simulink model "5kW_singlephase_grid-connected inverter_"  (R2020b)
settings: Solver=FixedStepDiscrete  StartTime=0.0  StopTime=10  FixedStep=1e-6  RelTol=1e-3
undefined symbols (not defined in the file): sigbuilder_block
libraries: powerlib x17, simulink x2, pid_lib x2, re_lib x1, powerlib_meascontrol x1
settings Model: SimulationMode=accelerator  Creator=zhaoy  LastModifiedBy=gc45
settings DataIOCC: ReturnWorkspaceOutputs=off
settings OptimizationCC: LifeSpan=inf
settings DebuggingCC: ArithmeticOperatorsInVariantConditions=warning
settings SFSimCC: SimUseLocalCustomCode=off  CustomCodeUndefinedFunction=UseInterfaceOnly
settings RTWCC: RTWUseLocalCustomCode=off
settings CodeAppCC: StateflowObjectComments=on
settings SimscapeCC: SimscapeNormalizeSystem=off

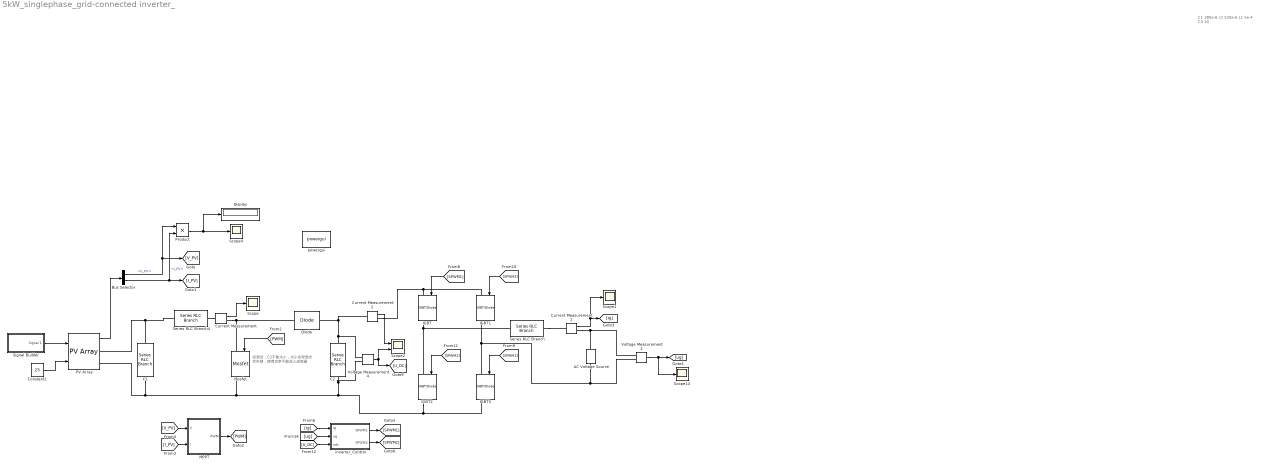
== system 5kW_singlephase_grid-connected inverter_ ==
  note: C1 380e-6
      | c2 520e-6
      | L1 5e-4
      | C3 20
  note: 经测试，C2不能太小，太小会导致光
      | 伏失稳，使得功率不能流入逆变器
  AC Voltage Source : powerlib/Electrical Sources/AC Voltage Source  Amplitude=311  Phase=180  Frequency=50  SampleTime=0  Measurements=None  BusType=swing  Pref=10e3  Qref=0  Qmin=-inf  Qmax=+inf
  Bus Selector : BusSelector  OutputSignals=V_PV,I_PV
  C1 : powerlib/Elements/Series RLC Branch  LConnTagsString=__new0  RConnTagsString=__new0  BranchType=C  Resistance=1  Inductance=3.05e-3  SetiL0=off  InitialCurrent=0  Capacitance=10e-6  Setx0=off  InitialVoltage=0  Measurements=Branch voltage
  C2 : powerlib/Elements/Series RLC Branch  LConnTagsString=__new0  RConnTagsString=__new0  BranchType=C  Resistance=1  Inductance=3.05e-3  SetiL0=off  InitialCurrent=0  Capacitance=6e-3  Setx0=off  InitialVoltage=0  Measurements=Branch voltage
  Constant1 : Constant  Value=25
  Current Measurement : powerlib/Measurements/Current Measurement  PhasorSimulation=off  OutputType=Complex  PSBequivalent=0
  Current Measurement1 : powerlib/Measurements/Current Measurement  PhasorSimulation=off  OutputType=Complex  PSBequivalent=0
  Current Measurement2 : powerlib/Measurements/Current Measurement  PhasorSimulation=off  OutputType=Complex  PSBequivalent=0
  Diode : powerlib/Power Electronics/Diode  Ron=0.001  Lon=0  Vf=0.8  IC=0  UseSnubber=off  Rs=500  Cs=250e-9  Measurements=off
  Display : Display
  IGBT{,1..3} (4 alike) : powerlib/Power Electronics/IGBT//Diode  Ron=1e-3  Rs=1e5  Cs=inf  Measurements=on
  MPPT : Subsystem
  Mosfet : powerlib/Power Electronics/Mosfet  Ron=0.1  Lon=0  Rd=0.01  Vfd=0  IC=0  Rs=1e5  Cs=inf  Measurements=on
  PV Array : re_lib/Solar/PV Array  Npar=2  Nser=7  PlotType=array @ 25 deg.C & specified irradiances  S_vec=[2000 1500 1000 ]  Temp_C_vec="[ 45 25  ]"  ModuleName=User-defined  PlotWhenSelected=off  Pm=213.15  Ncell=60  Voc=36.3  Isc=7.84  Vm=29  Im=7.35  beta_Voc_pc=-0.36099  alpha_Isc_pc=0.102  beta_Voc=-0.13104  alpha_Isc=0.0079968  IL=7.8654  I0=2.9273e-10  nI=0.98119  Rsh=313.0553  Rs=0.39381  RobustModel=off  RobustCellTemperature=313.3991  BAL=on  Tc=1e-6  Tfilter=5e-5
  Product : Product
  Scope{,1,4,14} (4 alike) : Scope
  Scope2 : Scope  NumInputPorts=2
  Series RLC Branch : powerlib/Elements/Series RLC Branch  LConnTagsString=__new0  RConnTagsString=__new0  BranchType=RL  Resistance=0.01  Inductance=20e-3  SetiL0=off  InitialCurrent=0  Capacitance=1e-6  Setx0=off  InitialVoltage=0  Measurements=None
  Series RLC Branch4 : powerlib/Elements/Series RLC Branch  LConnTagsString=__new0  RConnTagsString=__new0  BranchType=L  Resistance=1  Inductance=2.65e-3  SetiL0=off  InitialCurrent=0  Capacitance=1e-6  Setx0=off  InitialVoltage=0  Measurements=None
  Signal Builder : Subsystem  Tag=STV Subsys  LoadFcn=sigbuilder_block('load');  StartFcn=sigbuilder_block('start');  StopFcn=sigbuilder_block('stop');  ClipboardFcn=sigbuilder_block('clipboard');  mask(Sigbuilder block){tuvar=[0:10]}
      mask help: Simulink:masks:SigbuilderBlock_MD
      mask init:
      | if ~strcmp(get_param(bdroot(gcbh),'SimulationStatus'),'stopped') tuvar = sigbuilder_block('maskInit'); end
      settings: CopyFcn=sigbuilder_block('copy');  DeleteFcn=sigbuilder_block('delete');  ModelCloseFcn=sigbuilder_block('modelClose');  PreSaveFcn=sigbuilder_block('preSave');  PauseFcn=sigbuilder_block('pause');  ContinueFcn=sigbuilder_block('continue');  NameChangeFcn=sigbuilder_block('namechange');  OpenFcn=sigbuilder_block('open',[437.6 199.2 550.4 400 ]);  CloseFcn=sigbuilder_block('close');
      mask Display: plot(0, 0, 100, 100,[2, 2, 32, 32, 2], [68, 8, 8, 68, 68],[32, 2], [38, 38], [32, 19, 2],[53, 60, 44], [32, 17, 17, 2],[16, 16, 31, 31]);txt = getActiveGroup(gcbh);text(2, 100, txt,'verticalAlignment', 'top');
  Voltage Measurement2 : powerlib/Measurements/Voltage Measurement  PhasorSimulation=off  OutputType=Complex  PSBequivalent=0
  Voltage Measurement4 : powerlib/Measurements/Voltage Measurement  PhasorSimulation=off  OutputType=Complex  PSBequivalent=0
  inverter_Control : Subsystem
  powergui : powerlib/powergui  Priority=1  SimulationMode=Discrete  SampleTime=1e-6  frequency=50  Iterations=50  frequencyindice=0  Pbase=100e6  ErrMax=1e-4  UnitsV=kV  UnitsW=MW  buscounter=0  FunctionMessages=off  echomessages=off  EnableUseOfTLC=off  CurrentSourceSwitches=off  DisableSnubberDevices=off  DisableRonSwitches=off  DisableVfSwitches=off  DisplayEquations=off  AutomaticDiscreteSolvers=off  SolverType=Tustin/Backward Euler (TBE)  Interpol=off  ExternalGateDelay=off  methode=off  Ts=10  x0status=blocks  SPID=off  SwTol=0  HookPort=off  NonlinearTolerance=1e-4  nMaxIteration=100  ContinueOnMaxIteration=off  RestoreLinks=warning  ResistiveCurrentMeasurement=off  Frange=[0:2:500]  Ylog=off  Xlog=on  ShowGrid=off  save=off  variable=ZData  structure=Udc_pv  ZoomFFT=off  StartTime=8  cycles=20  DisplayStyle=1  fundamental=50  FreqAxis=on  MaxFrequency=500  frequencyindicesteady=1  RmsSteady=2  display=off
  wires:
  PV Array/1 -> Bus Selector/1
  [PWM] -> Mosfet/1
  Signal Builder/1(Signal 1) -> PV Array/1
  Constant1/1 -> PV Array/2
  Bus Selector/1 -> Product/1, [V_PV]  "<V_PV>"
  Bus Selector/2 -> Product/2, [I_PV]  "<I_PV>"
  Product/1 -> Display/1, Scope4/1
  [V_PV] -> MPPT/1(V)
  [I_PV] -> MPPT/2(I)
  MPPT/1(PWM) -> [PWM]
  Current Measurement1/1 -> Scope1/1, [ig]
  Voltage Measurement2/1 -> Scope14/1, [ug]
  [SPWM1] -> IGBT/1
  [SPWM1] -> IGBT3/1
  [SPWM2] -> IGBT1/1
  [SPWM2] -> IGBT2/1
  Current Measurement/1 -> Scope/1
  Voltage Measurement4/1 -> Scope2/2, [U_DC]
  Current Measurement2/1 -> Scope2/1
  [ig] -> inverter_Control/1(Ig)
  [ug] -> inverter_Control/2(ug)
  [U_DC] -> inverter_Control/3(udc)
  inverter_Control/1(SPWM1) -> [SPWM1]
  inverter_Control/2(SPWM2) -> [SPWM2]
  connections:
  IGBT2/LConn1 -- Series RLC Branch/LConn1 -- IGBT/RConn1
  IGBT3/LConn1 -- IGBT1/RConn1 -- Voltage Measurement2/LConn2 -- AC Voltage Source/RConn1
  Current Measurement/RConn1 -- Mosfet/LConn1 -- Diode/LConn1
  C1/LConn1 -- Series RLC Branch4/LConn1 -- PV Array/RConn1
  IGBT2/RConn1 -- PV Array/RConn2 -- C1/RConn1 -- Mosfet/RConn1 -- Voltage Measurement4/LConn2 -- C2/RConn1 -- IGBT3/RConn1
  Current Measurement1/RConn1 -- Voltage Measurement2/LConn1 -- AC Voltage Source/LConn1
  Series RLC Branch4/RConn1 -- Current Measurement/LConn1
  Series RLC Branch/RConn1 -- Current Measurement1/LConn1
  Voltage Measurement4/LConn1 -- Current Measurement2/LConn1 -- Diode/RConn1 -- C2/LConn1
  IGBT1/LConn1 -- Current Measurement2/RConn1 -- IGBT/LConn1

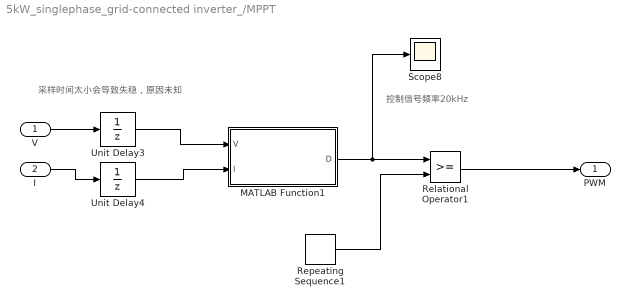
== system 5kW_singlephase_grid-connected inverter_/MPPT ==
  note: 采样时间太小会导致失稳，原因未知
  note: 控制信号频率20kHz
  V : Inport
  I : Inport  Port=2
  MATLAB Function1 : MATLAB Function  TreatAsAtomicUnit=on
  Relational Operator1 : RelationalOperator  OutDataTypeStr=boolean  RndMeth=Nearest
  Repeating Sequence1 : simulink/Sources/Repeating Sequence  rep_seq_t=[0 1/20000]  rep_seq_y=[0 1]
  Scope8 : Scope
  Unit Delay3 : UnitDelay  SampleTime=1e-4  HasFrameUpgradeWarning=on
  Unit Delay4 : UnitDelay  SampleTime=1e-4  HasFrameUpgradeWarning=on
  PWM : Outport
  wires:
  I/1 -> Unit Delay4/1
  V/1 -> Unit Delay3/1
  Relational Operator1/1 -> PWM/1
  Repeating Sequence1/1 -> Relational Operator1/2
  MATLAB Function1/1(D) -> Scope8/1, Relational Operator1/1
  Unit Delay3/1 -> MATLAB Function1/1(V)
  Unit Delay4/1 -> MATLAB Function1/2(I)

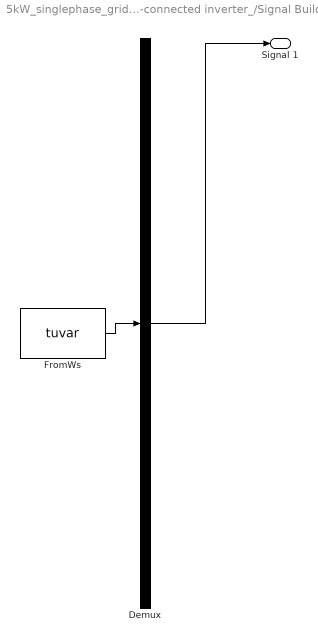
== system 5kW_singlephase_grid-connected inverter_/Signal Builder ==
  Demux : Demux  Tag=STV Demux  Outputs=1
      settings: DisplayOption=none
  FromWs : FromWorkspace  Tag=STV FromWs  VariableName=tuvar
      SigBuilderData=|
      | common.afterFinalStr = 'Extrapolate'
      | common.sampleTime = 0
      | dataSet.timeRange = [0 10]
      | dataSet.name = 'Group 1'
      | sbobj.Groups.Name = 'Group 1'
      | sbobj.Groups.Signals.Name = 'Signal 1'
      | sbobj.Groups.Signals.XData = [0 3 3 5 5 10]
      | sbobj.Groups.Signals.YData = [2000 2000 1500 1500 1000 1000]
  Signal 1 : Outport  Tag=STV Outport
  wires:
  Demux/1 -> Signal 1/1
  FromWs/1 -> Demux/1

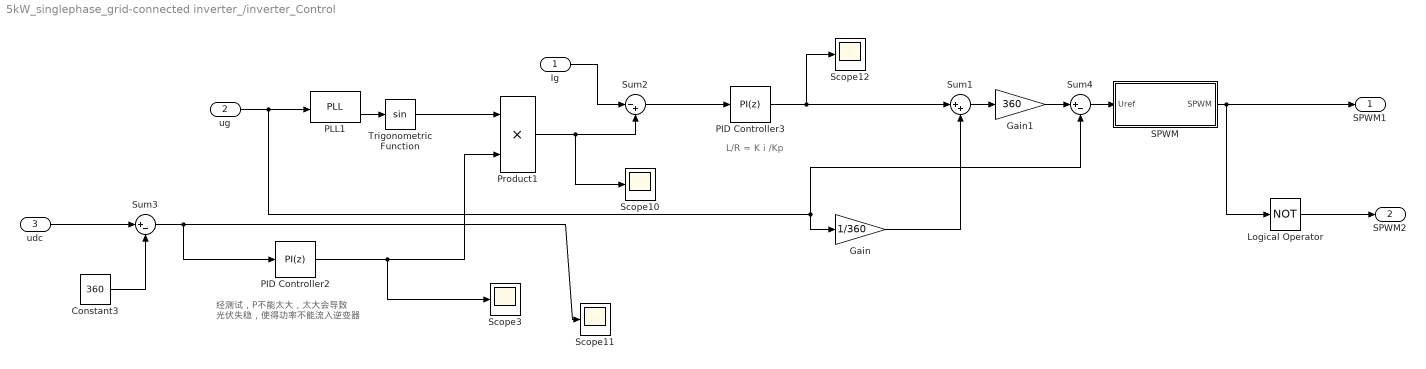
== system 5kW_singlephase_grid-connected inverter_/inverter_Control ==
  note: 经测试，P不能太大，太大会导致
      | 光伏失稳，使得功率不能流入逆变器
  note: L/R = K i /Kp
  Ig : Inport
  ug : Inport  Port=2
  udc : Inport  Port=3
  Constant3 : Constant  Value=360
  Gain : Gain  Gain=1/360
  Gain1 : Gain  Gain=360
  Logical Operator : Logic  Operator=NOT  AllPortsSameDT=off  OutDataTypeStr=boolean
  PID Controller2 : pid_lib/PID Controller  Controller=PI  Form=Parallel  TimeDomain=Discrete-time  UseExternalTs=off  SampleTime=-1  IntegratorMethod=Forward Euler  FilterMethod=Forward Euler  ControllerParametersSource=internal  P=0.1  I=1.5  D=0  UseFilter=on  N=100  TunerSelectOption=Transfer Function Based (PID Tuner App)  InitialConditionSource=internal  InitialConditionForIntegrator=0  InitialConditionForFilter=0  DifferentiatorICPrevScaledInput=0  ExternalReset=none  TrackingMode=off  Kt=1  LimitOutput=off  SatLimitsSource=internal  UpperSaturationLimit=1  LowerSaturationLimit=-1  LinearizeAsGain=on  AntiWindupMode=none  Kb=1  POutMin=[]  POutMax=[]  IOutMin=[]  IOutMax=[]  DOutMin=[]  DOutMax=[]  NOutMin=[]  NOutMax=[]  SumOutMin=[]  SumOutMax=[]  SaturationOutMin=[]  SaturationOutMax=[]  PParamMin=[]  PParamMax=[]  IParamMin=[]  IParamMax=[]  DParamMin=[]  DParamMax=[]  NParamMin=[]  NParamMax=[]  KbParamMin=[]  KbParamMax=[]  KtParamMin=[]  KtParamMax=[]  KbOutMin=[]  KbOutMax=[]  KtOutMin=[]  KtOutMax=[]  IntegratorOutMin=[]  IntegratorOutMax=[]  FilterOutMin=[]  FilterOutMax=[]  SumI1OutMin=[]  SumI1OutMax=[]  SumI2OutMin=[]  SumI2OutMax=[]  SumI3OutMin=[]  SumI3OutMax=[]  SumI4OutMin=[]  SumI4OutMax=[]  SumDOutMin=[]  SumDOutMax=[]  DifferentiatorOutMin=[]  DifferentiatorOutMax=[]  FilterDiffOutCoefMin=[]  FilterDiffOutCoefMax=[]  ReciprocalOutMin=[]  ReciprocalOutMax=[]  SumDenOutMin=[]  SumDenOutMax=[]  SumNumOutMin=[]  SumNumOutMax=[]  DivideOutMin=[]  DivideOutMax=[]  UdiffTsProdOutMin=[]  UdiffTsProdOutMax=[]  NTsProdOutMin=[]  NTsProdOutMax=[]  UintegralTsProdOutMin=[]  UintegralTsProdOutMax=[]  UngainTsProdOutMin=[]  UngainTsProdOutMax=[]  IntegratorContinuousStateAttributes=''  IntegratorStateMustResolveToSignalObject=off  IntegratorRTWStateStorageClass=Auto  FilterContinuousStateAttributes=''  FilterStateMustResolveToSignalObject=off  FilterRTWStateStorageClass=Auto  ParallelPVariant=InternalParameters  IdealPVariant=Disabled  IVariant=InternalParameters  DVariant=Disabled  IntegratorVariant=Discrete  SatVariant=Disabled  AWVariant=Passthrough  PCopyVariant=Disabled  TRVariant=Disabled  FdbkBlocksVariant=Forward  IdealPFdbkVariant=Disabled  SatFdbkVariant=Disabled  DerivativeFilterVariant=Disabled  NVariant=Disabled  NCopyVariant=Disabled_SignalSpec  FilterICVariant=Disabled  IntegratorICVariant=InternalICs  ExternalResetVariant=Disabled  TRSumVariant=Passthrough  SumFdbkVariant=Disabled  SumVariant=Sum_PI  TsampFilterVariant=InternalTs  TsampNgainVariant=Passthrough  TsampIntegralVariant=Passthrough  ExternalSaturationOutDataTypeStr=Inherit: Same as second input
  PID Controller3 : pid_lib/PID Controller  Controller=PI  Form=Parallel  TimeDomain=Discrete-time  UseExternalTs=off  SampleTime=-1  IntegratorMethod=Forward Euler  FilterMethod=Forward Euler  ControllerParametersSource=internal  P=10  I=20  D=0  UseFilter=on  N=100  TunerSelectOption=Transfer Function Based (PID Tuner App)  InitialConditionSource=internal  InitialConditionForIntegrator=0  InitialConditionForFilter=0  DifferentiatorICPrevScaledInput=0  ExternalReset=none  TrackingMode=off  Kt=1  LimitOutput=off  SatLimitsSource=internal  UpperSaturationLimit=1  LowerSaturationLimit=-1  LinearizeAsGain=on  AntiWindupMode=none  Kb=1  POutMin=[]  POutMax=[]  IOutMin=[]  IOutMax=[]  DOutMin=[]  DOutMax=[]  NOutMin=[]  NOutMax=[]  SumOutMin=[]  SumOutMax=[]  SaturationOutMin=[]  SaturationOutMax=[]  PParamMin=[]  PParamMax=[]  IParamMin=[]  IParamMax=[]  DParamMin=[]  DParamMax=[]  NParamMin=[]  NParamMax=[]  KbParamMin=[]  KbParamMax=[]  KtParamMin=[]  KtParamMax=[]  KbOutMin=[]  KbOutMax=[]  KtOutMin=[]  KtOutMax=[]  IntegratorOutMin=[]  IntegratorOutMax=[]  FilterOutMin=[]  FilterOutMax=[]  SumI1OutMin=[]  SumI1OutMax=[]  SumI2OutMin=[]  SumI2OutMax=[]  SumI3OutMin=[]  SumI3OutMax=[]  SumI4OutMin=[]  SumI4OutMax=[]  SumDOutMin=[]  SumDOutMax=[]  DifferentiatorOutMin=[]  DifferentiatorOutMax=[]  FilterDiffOutCoefMin=[]  FilterDiffOutCoefMax=[]  ReciprocalOutMin=[]  ReciprocalOutMax=[]  SumDenOutMin=[]  SumDenOutMax=[]  SumNumOutMin=[]  SumNumOutMax=[]  DivideOutMin=[]  DivideOutMax=[]  UdiffTsProdOutMin=[]  UdiffTsProdOutMax=[]  NTsProdOutMin=[]  NTsProdOutMax=[]  UintegralTsProdOutMin=[]  UintegralTsProdOutMax=[]  UngainTsProdOutMin=[]  UngainTsProdOutMax=[]  IntegratorContinuousStateAttributes=''  IntegratorStateMustResolveToSignalObject=off  IntegratorRTWStateStorageClass=Auto  FilterContinuousStateAttributes=''  FilterStateMustResolveToSignalObject=off  FilterRTWStateStorageClass=Auto  ParallelPVariant=InternalParameters  IdealPVariant=Disabled  IVariant=InternalParameters  DVariant=Disabled  IntegratorVariant=Discrete  SatVariant=Disabled  AWVariant=Passthrough  PCopyVariant=Disabled  TRVariant=Disabled  FdbkBlocksVariant=Forward  IdealPFdbkVariant=Disabled  SatFdbkVariant=Disabled  DerivativeFilterVariant=Disabled  NVariant=Disabled  NCopyVariant=Disabled_SignalSpec  FilterICVariant=Disabled  IntegratorICVariant=InternalICs  ExternalResetVariant=Disabled  TRSumVariant=Passthrough  SumFdbkVariant=Disabled  SumVariant=Sum_PI  TsampFilterVariant=InternalTs  TsampNgainVariant=Passthrough  TsampIntegralVariant=Passthrough  ExternalSaturationOutDataTypeStr=Inherit: Same as second input
  PLL1 : powerlib_meascontrol/PLL/PLL  Fmin=45  Par_Init=[0 50]  ParK=[1,20]  TcD=5e-6  MaxRateChangeFreq=12  FilterCutOffFreq=25  Ts=1e-6  AGC=on
      settings: SourceProductBaseCode=PS
  Product1 : Product
  SPWM : Subsystem
  Scope{3,10..12} (4 alike) : Scope
  Sum1 : Sum  Inputs=|++
  Sum2 : Sum  Inputs=|-+
  Sum3 : Sum  Inputs=|+-
  Sum4 : Sum  Inputs=|+-
  Trigonometric Function : Trigonometry
  SPWM1 : Outport
  SPWM2 : Outport  Port=2
  wires:
  Constant3/1 -> Sum3/2
  Sum2/1 -> PID Controller3/1
  ug/1 -> Gain/1, Sum4/2, PLL1/1
  Sum4/1 -> SPWM/1(Uref)
  SPWM/1(SPWM) -> SPWM1/1, Logical Operator/1
  Trigonometric Function/1 -> Product1/1
  Gain1/1 -> Sum4/1
  PLL1/2 -> Trigonometric Function/1
  PID Controller2/1 -> Scope3/1, Product1/2
  Sum1/1 -> Gain1/1
  Product1/1 -> Scope10/1, Sum2/2
  PID Controller3/1 -> Sum1/1, Scope12/1
  Sum3/1 -> PID Controller2/1, Scope11/1
  Gain/1 -> Sum1/2
  Logical Operator/1 -> SPWM2/1
  udc/1 -> Sum3/1
  Ig/1 -> Sum2/1

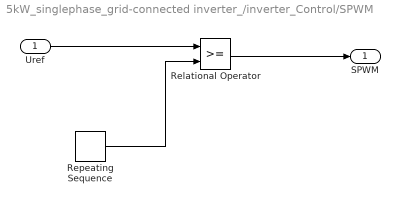
== system 5kW_singlephase_grid-connected inverter_/inverter_Control/SPWM ==
  Uref : Inport
  Relational Operator : RelationalOperator  OutDataTypeStr=boolean  RndMeth=Nearest
  Repeating Sequence : simulink/Sources/Repeating Sequence  rep_seq_t=[0 0.0000125 0.0000375 0.00005]  rep_seq_y=[0 -1 1 0]
  SPWM : Outport
  wires:
  Uref/1 -> Relational Operator/1
  Relational Operator/1 -> SPWM/1
  Repeating Sequence/1 -> Relational Operator/2

== matlab function 5kW_singlephase_grid-connected inverter_/MPPT/MATLAB Function1 ==
  data: V input; D output; I input

function D=DutyRatio(V,I)

Dmax=0.95;
Dmin=0.0;
Dinit=0.5;
deltaD=0.001;
persistent Vold Pold Dold;

dataType = 'double';


if isempty(Vold)
	Vold=0;
	Pold=0;
	Dold=Dinit;
end

p=V*I;
dV=V-Vold;
dp=p-Pold;

if dp~=0
	if dp<0
		if dV<0
			D=Dold-deltaD;
		else
			D=Dold+deltaD;
		end
	else
		if dV< 0
			D=Dold+deltaD;
		else
			D=Dold-deltaD;
		end
	end
else
    D=Dold;
end

if D>=Dmax || D<=Dmin
	D=Dold;
end

Dold=D;
Vold=V;
Pold=p;
